simulink model "abs_core"  (R2024b)
settings: Solver=VariableStepAuto  StartTime=0.0  StopTime=10.0  RelTol=1e-3
undefined symbols (not defined in the file or in its folder): PAR_TIRE_d_RollingRadius
settings Model: Creator=rocke  LastModifiedBy=rocke
settings DataIOCC: SaveState=on

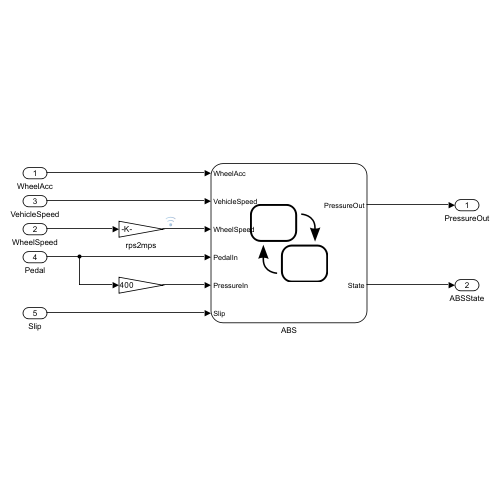
[thumbnail: Simulink's stored preview of the top-level diagram]
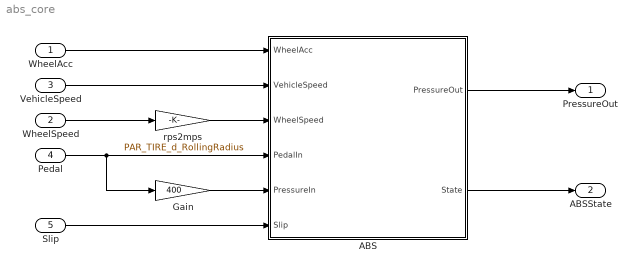
== system abs_core ==
  WheelAcc : Inport
  WheelSpeed : Inport  Port=2  Unit=rad/s
  VehicleSpeed : Inport  Port=3  Unit=m/s
  Pedal : Inport  Port=4
  Slip : Inport  Port=5
  ABS : Stateflow chart  TreatAsAtomicUnit=on
  Gain : Gain  Gain=400
  rps2mps : Gain  Gain=PAR_TIRE_d_RollingRadius
  PressureOut : Outport
  ABSState : Outport  Port=2
  wires:
  WheelAcc/1 -> ABS/1(WheelAcc)
  VehicleSpeed/1 -> ABS/2(VehicleSpeed)
  WheelSpeed/1 -> rps2mps/1
  Pedal/1 -> Gain/1, ABS/4(PedalIn)
  Gain/1 -> ABS/5(PressureIn)
  rps2mps/1 -> ABS/3(WheelSpeed)
  ABS/2(State) -> ABSState/1
  ABS/1(PressureOut) -> PressureOut/1
  Slip/1 -> ABS/6(Slip)

== stateflow chart abs_core/ABS ==
  settings: updateMethod=DISCRETE  sampleTime=1e-2
  state Active
    state Increase
      du: PressureOut = min(PressureIn, PressureOut + 20);
    state Drop
      du: PressureOut = max(0, PressureOut - 25.0);
    (default) -> Increase
    Drop -> Increase : [abs(Slip) < 0.15 || ...
        | WheelAcc > 10]
    Increase -> Drop : [abs(Slip) > 0.25 || ...
        | WheelAcc < -100]
  state Inactive
    en: PressureOut = 0;
  state Passive
    en: PressureOut = PressureIn;
    du: PressureOut = PressureIn;
  (default) -> Inactive
  Inactive -> Passive : [PedalIn > 0.02]
  Passive -> Inactive [order 1] : [PedalIn < 0.02]
  Passive -> Active [order 2] : [(0.8 < PedalIn || ...
      | WheelAcc < -100) && ...
      | VehicleSpeed >= 1 ]
  Active -> Passive : [VehicleSpeed < 1]
  data: WheelAcc input; VehicleSpeed input; WheelSpeed input; PedalIn input; PressureIn input; PressureOut output [..10]; State output Enum: ChartModeType; Pressure local; Slip input
